simulink model "Control"  (R2022b)
settings: Solver=FixedStepDiscrete  StartTime=0.0  StopTime=inf  FixedStep=Ts  RelTol=1e-3
undefined symbols (not defined in the file): Ts
libraries: robotalgslib x1
settings Model: Creator=mluo  LastModifiedBy=mluo
settings DataIOCC: SaveOutput=off  SaveTime=off
settings OptimizationCC: DefaultParameterBehavior=Inlined  EnhancedBackFolding=on  PassReuseOutputArgsAs=Individual arguments  ZeroExternalMemoryAtStartup=off  ZeroInternalMemoryAtStartup=off  MaxStackSize=64  OptimizeBlockOrder=speed  DifferentSizesBufferReuse=on  OptimizationCustomize=off  EfficientTunableParamExpr=on
settings DebuggingCC: ParameterTunabilityLossMsg=error  UnconnectedInputMsg=warning  UnconnectedOutputMsg=warning  UnconnectedLineMsg=warning
settings ModelReferenceCC: EnableRefExpFcnMdlSchedulingChecks=on
settings SFSimCC: MATLABDynamicMemAlloc=off
settings RTWCC: Description=Embedded Coder  SystemTargetFile=ert.tlc  GenCodeOnly=on  TemplateMakefile=ert_default_tmf  BuildConfiguration=Faster Runs  DLArmComputeVersion=19.05
settings CodeAppCC: ForceParamTrailComments=on  IgnoreCustomStorageClasses=off  OperatorAnnotations=on  SimulinkDataObjDesc=on  SFDataObjDesc=on  InsertBlockDesc=on
settings ERTTargetCC: GenerateSampleERTMain=on  InlinedParameterPlacement=NonHierarchical  ERTCustomFileTemplate=example_file_process.tlc
settings ConfigComp: PSVerificationMode=BugFinder  PSOpenProjectManager=on  PSAutoStubLUT=on

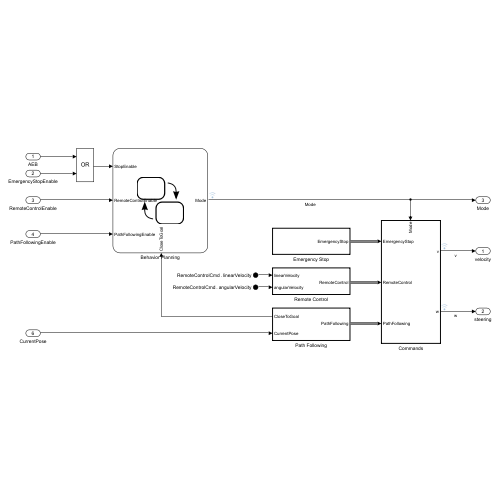
[thumbnail: Simulink's stored preview of the top-level diagram]
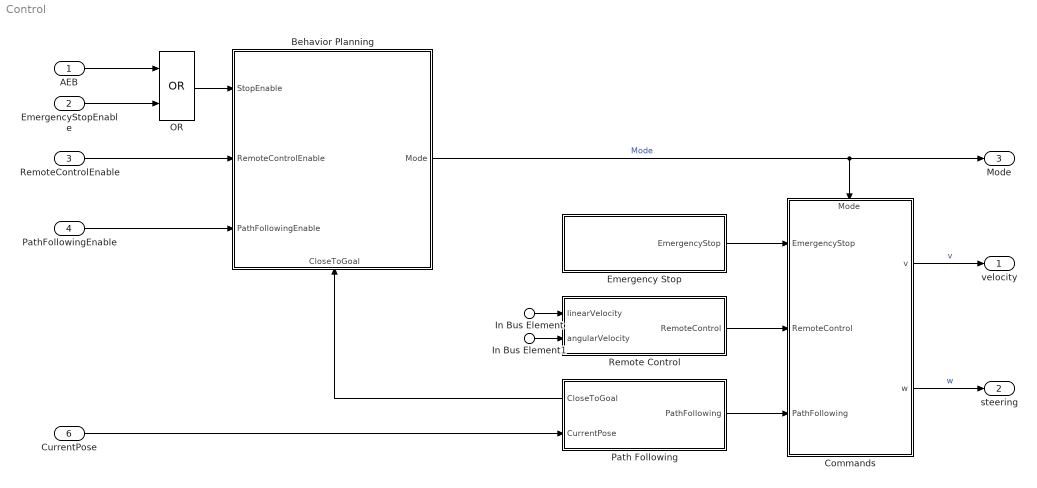
== system Control ==
  AEB : Inport  OutDataTypeStr=boolean  PortDimensions=1  SampleTime=Ts
  EmergencyStopEnable : Inport  Port=2  OutDataTypeStr=boolean  PortDimensions=1  SampleTime=Ts
  RemoteControlEnable : Inport  Port=3  OutDataTypeStr=boolean  PortDimensions=1  SampleTime=Ts
  PathFollowingEnable : Inport  Port=4  OutDataTypeStr=boolean  PortDimensions=1  SampleTime=Ts
  In Bus Element : Inport  Port=5  PortName=RemoteControlCmd  Element=linearVelocity
  In Bus Element1 : Inport  Port=5  PortName=RemoteControlCmd  Element=angularVelocity
  CurrentPose : Inport  Port=6  OutDataTypeStr=double  PortDimensions=3  SampleTime=Ts
  Behavior Planning : Stateflow chart  TreatAsAtomicUnit=on
      settings: PortSchema="{\"entries\":[{\"content\":{\"sides\":[{\"content\":{\"connectorIds\":[\"In4\",\"In2\",\"In3\"]},\"type\":\"ConnectorPlacement.EquallySpacedRectSide\",\"uuid\":\"c24f9a90-a87f-41b0-b779-13c2bcfc899f\"},{\"content\":{\"connectorIds\":[\"Out1\"],\"side\":\"RIGHT\"},\"type\":\"ConnectorPlacement.EquallySpacedRectSide\",\"uuid\":\"043f7b90-2386-4dc9-846f-9317a0a81ec4\"},{\"content\":{\"connectorIds\":[],\"side\":\"TOP\"},\"type\":\"ConnectorPlacement.EquallySpacedRectSide\",\"uuid\":\"89f6e0a0-964d-4138-9fcf-6abccaea390e\"},{\"content\":{\"connectorIds\":[\"In1\"],\"side\":\"BOTTOM\"},\"type\":\"ConnectorPlacement.EquallySpacedRectSide\",\"uuid\":\"8e73b273-e6b3-46d9-b7e2-d7b7e94549f0\"}]},\"type\":\"ConnectorPlacement.EquallySpacedConnector\",\"uuid\":\"e375211d-348b-4057-bdf9-d0981c9d3a60\"}],\"packageUris\":[\"http://schema.mathworks.com/mf0/Connector/R2020b\"],\"version\":\"1.0\"}"
  Commands : Subsystem  TreatAsAtomicUnit=on
      settings: PortSchema="{\"entries\":[{\"content\":{\"sides\":[{\"content\":{\"connectorIds\":[\"In1\",\"In2\",\"In3\"]},\"type\":\"ConnectorPlacement.EquallySpacedRectSide\",\"uuid\":\"0a16c418-6526-4a2f-9b2d-354d66f674c4\"},{\"content\":{\"connectorIds\":[\"Out1\",\"Out2\"],\"side\":\"RIGHT\"},\"type\":\"ConnectorPlacement.EquallySpacedRectSide\",\"uuid\":\"f4f8e36b-1e4f-40f2-b6fc-cacf05e58e0d\"},{\"content\":{\"connectorIds\":[\"In4\"],\"side\":\"TOP\"},\"type\":\"ConnectorPlacement.EquallySpacedRectSide\",\"uuid\":\"de2c763d-2057-494d-a303-a24b01099b3b\"}]},\"type\":\"ConnectorPlacement.EquallySpacedConnector\",\"uuid\":\"58b52408-98ad-46e9-802c-d15590c77517\"}],\"packageUris\":[\"http://schema.mathworks.com/mf0/Connector/R2020b\"],\"version\":\"1.0\"}"
  Emergency Stop : Subsystem  TreatAsAtomicUnit=on
  OR : Logic  Operator=OR  AllPortsSameDT=off  OutDataTypeStr=boolean
  Path Following : Subsystem  TreatAsAtomicUnit=on
      settings: PortSchema="{\"entries\":[{\"content\":{\"sides\":[{\"content\":{\"connectorIds\":[\"Out2\",\"In1\"]},\"type\":\"ConnectorPlacement.EquallySpacedRectSide\",\"uuid\":\"51024eaf-60b5-4ae4-a60b-2aa0725bc647\"},{\"content\":{\"connectorIds\":[\"Out1\"],\"side\":\"RIGHT\"},\"type\":\"ConnectorPlacement.EquallySpacedRectSide\",\"uuid\":\"f8f735f7-4a82-46fe-95f3-240be1725304\"},{\"content\":{\"connectorIds\":[],\"side\":\"TOP\"},\"type\":\"ConnectorPlacement.EquallySpacedRectSide\",\"uuid\":\"a6f2919d-39bb-452c-95b9-5a0efbd40615\"},{\"content\":{\"connectorIds\":[],\"side\":\"BOTTOM\"},\"type\":\"ConnectorPlacement.EquallySpacedRectSide\",\"uuid\":\"68f6689d-e8c4-4f54-9215-202253622632\"}]},\"type\":\"ConnectorPlacement.EquallySpacedConnector\",\"uuid\":\"e8a362bf-3ecd-4ba6-82c8-3e5a3b2b329c\"}],\"packageUris\":[\"http://schema.mathworks.com/mf0/Connector/R2020b\"],\"version\":\"1.0\"}"
  Remote Control : Subsystem  TreatAsAtomicUnit=on
  velocity : Outport  OutDataTypeStr=double  PortDimensions=1  SampleTime=Ts
  steering : Outport  Port=2  OutDataTypeStr=double  PortDimensions=1  SampleTime=Ts
  Mode : Outport  Port=3  OutDataTypeStr=int32  PortDimensions=1  SampleTime=Ts
  wires:
  Path Following/1(PathFollowing) -> Commands/3(PathFollowing)
  PathFollowingEnable/1 -> Behavior Planning/3(PathFollowingEnable)
  Behavior Planning/1(Mode) -> Commands/4(Mode), Mode/1  "Mode"
  Commands/2(w) -> steering/1  "w"
  Remote Control/1(RemoteControl) -> Commands/2(RemoteControl)
  Emergency Stop/1(EmergencyStop) -> Commands/1(EmergencyStop)
  Path Following/2(CloseToGoal) -> Behavior Planning/1(CloseToGoal)
  CurrentPose/1 -> Path Following/1(CurrentPose)
  RemoteControlEnable/1 -> Behavior Planning/2(RemoteControlEnable)
  Commands/1(v) -> velocity/1  "v"
  In Bus Element/1 -> Remote Control/1(linearVelocity)
  In Bus Element1/1 -> Remote Control/2(angularVelocity)
  OR/1 -> Behavior Planning/4(StopEnable)
  AEB/1 -> OR/1
  EmergencyStopEnable/1 -> OR/2

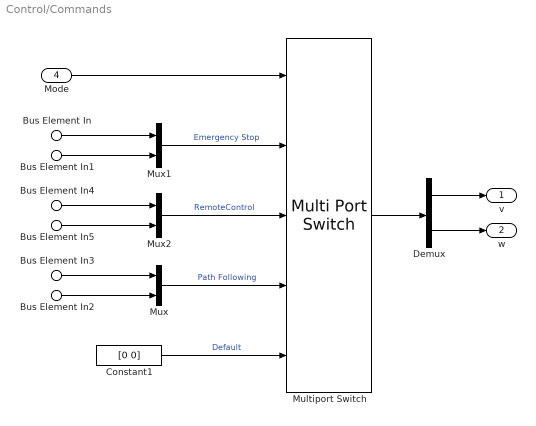
== system Control/Commands ==
  Bus Element In : Inport  PortName=EmergencyStop  Element=linearVelocity
  Bus Element In1 : Inport  PortName=EmergencyStop  Element=angularVelocity
  Bus Element In4 : Inport  Port=2  PortName=RemoteControl  Element=linearVelocity
  Bus Element In5 : Inport  Port=2  PortName=RemoteControl  Element=angularVelocity
  Bus Element In2 : Inport  Port=3  PortName=PathFollowing  Element=angularVelocity
  Bus Element In3 : Inport  Port=3  PortName=PathFollowing  Element=linearVelocity
  Mode : Inport  Port=4
  Constant1 : Constant  Value=[0 0]
  Demux : Demux  Outputs=2
  Multiport Switch : MultiPortSwitch  DataPortOrder=Zero-based contiguous  Inputs=4  zeroidx=on  SaturateOnIntegerOverflow=off  InputSameDT=off
  Mux : Mux  Inputs=2
  Mux1 : Mux  Inputs=2
  Mux2 : Mux  Inputs=2
  v : Outport
  w : Outport  Port=2
  wires:
  Mux2/1 -> Multiport Switch/3  "RemoteControl"
  Bus Element In5/1 -> Mux2/2
  Bus Element In4/1 -> Mux2/1
  Bus Element In/1 -> Mux1/1
  Bus Element In1/1 -> Mux1/2
  Demux/2 -> w/1
  Demux/1 -> v/1
  Multiport Switch/1 -> Demux/1
  Mux/1 -> Multiport Switch/4  "Path Following"
  Bus Element In2/1 -> Mux/2
  Bus Element In3/1 -> Mux/1
  Constant1/1 -> Multiport Switch/5  "Default"
  Mux1/1 -> Multiport Switch/2  "Emergency Stop"
  Mode/1 -> Multiport Switch/1

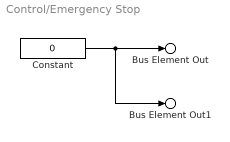
== system Control/Emergency Stop ==
  Constant : Constant  Value=0
  Bus Element Out : Outport  PortName=EmergencyStop  Element=linearVelocity
  Bus Element Out1 : Outport  PortName=EmergencyStop  Element=angularVelocity
  wires:
  Constant/1 -> Bus Element Out/1, Bus Element Out1/1

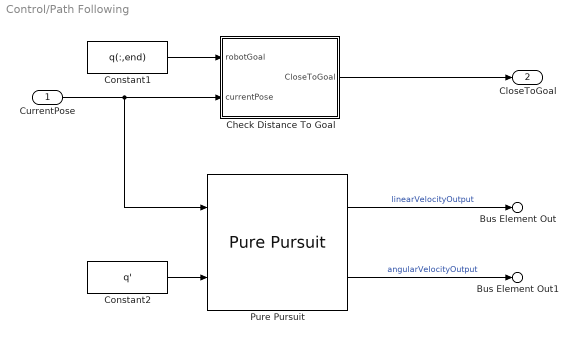
== system Control/Path Following ==
  CurrentPose : Inport
  Check Distance To Goal : Subsystem
  Constant1 : Constant  Value=q(:,end)
  Constant2 : Constant  Value=q'
  Pure Pursuit : robotalgslib/Pure Pursuit  DesiredLinearVelocity=5  MaxAngularVelocity=2  LookaheadDistance=2  TargetDirPort=off  SimulateUsing=Code generation
  Bus Element Out : Outport  PortName=PathFollowing  Element=linearVelocity
  Bus Element Out1 : Outport  PortName=PathFollowing  Element=angularVelocity
  CloseToGoal : Outport  Port=2
  wires:
  Constant2/1 -> Pure Pursuit/2
  Pure Pursuit/2 -> Bus Element Out1/1  "angularVelocityOutput"
  Pure Pursuit/1 -> Bus Element Out/1  "linearVelocityOutput"
  CurrentPose/1 -> Pure Pursuit/1, Check Distance To Goal/2(currentPose)
  Constant1/1 -> Check Distance To Goal/1(robotGoal)
  Check Distance To Goal/1(CloseToGoal) -> CloseToGoal/1

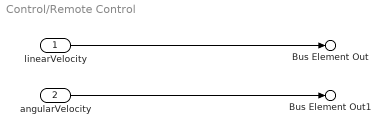
== system Control/Remote Control ==
  linearVelocity : Inport
  angularVelocity : Inport  Port=2
  Bus Element Out : Outport  PortName=RemoteControl  Element=linearVelocity
  Bus Element Out1 : Outport  PortName=RemoteControl  Element=angularVelocity
  wires:
  angularVelocity/1 -> Bus Element Out1/1
  linearVelocity/1 -> Bus Element Out/1

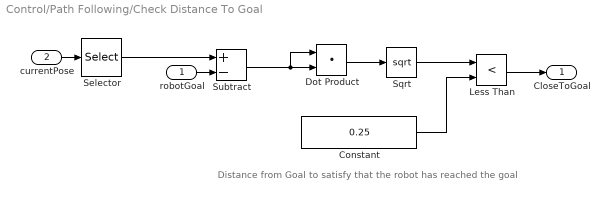
== system Control/Path Following/Check Distance To Goal ==
  note: Distance from Goal to satisfy that the robot has reached the goal
  robotGoal : Inport
  currentPose : Inport  Port=2
  Constant : Constant  Value=0.25
  Dot Product : DotProduct  OutDataTypeStr=Inherit: Inherit via internal rule
  Less Than : RelationalOperator  Operator=<  OutDataTypeStr=boolean  RndMeth=Simplest  InputSameDT=off
  Selector : Selector  InputPortWidth=3  IndexOptions=Index vector (dialog)  Indices=[1 2]  OutputSizes=1
  Sqrt : Sqrt
  Subtract : Sum  Inputs=+-
  CloseToGoal : Outport
  wires:
  Selector/1 -> Subtract/1
  Subtract/1 -> Dot Product/2, Dot Product/1
  Sqrt/1 -> Less Than/1
  Less Than/1 -> CloseToGoal/1
  currentPose/1 -> Selector/1
  Constant/1 -> Less Than/2
  Dot Product/1 -> Sqrt/1
  robotGoal/1 -> Subtract/2

== stateflow chart Control/Behavior Planning ==
  state Stop
    en:
    Mode = 0;
  state RemoteControl
    en:
    Mode = 1;
  state PathFollowing
    en:
    Mode = 2;
  (default) -> Stop : {Mode = 0;}
  (junction 12) -> Stop
  (junction 11) -> (junction 12)
  Stop -> Stop [order 1] : [StopEnable]
  (junction 20) -> Stop
  PathFollowing -> (junction 20) [order 1] : [StopEnable]
  Stop -> (junction 23) [order 3] : [PathFollowingEnable...
      | && ~CloseToGoal]
  (junction 23) -> PathFollowing
  RemoteControl -> Stop [order 1] : [StopEnable...
      | || ~RemoteControlEnable]
  Stop -> RemoteControl [order 2] : [RemoteControlEnable]
  RemoteControl -> PathFollowing [order 3] : [PathFollowingEnable]
  RemoteControl -> RemoteControl [order 2] : [RemoteControlEnable]
  PathFollowing -> (junction 11) [order 2] : [CloseToGoal...
      | || ~PathFollowingEnable]
  PathFollowing -> RemoteControl [order 3] : [RemoteControlEnable]
  data: CloseToGoal input; RemoteControlEnable input boolean; PathFollowingEnable input boolean; Mode output int32; StopEnable input
